simulink model "simulink_tirocinio3"  (R2021a)
settings: Solver=VariableStepAuto  StartTime=0.0  StopTime=100  RelTol=1e-3
values from neighbouring files (symbols this model uses):
  A = [lambda_1 0; 0 lambda_2]    [tirocinio1.m]    (also in tirocinio2.m = [0 1; gamma_1 gamma_2]; tirocinio3_complessiconiugati.m = [0 0 1 0; 0 0 0 1; -k_m/m1_m k_m/m1_m -c_m/m1_m c_m/m1_m; k_; tirocinio3_immaginari_puri.m = [0 0 1 0; 0 0 0 1; -k_m/m1_m k_m/m1_m -c_m/m1_m c_m/m1_m; k_; tirocinio3_reali.m = [0 0 1 0; 0 0 0 1; -k_m/m1_m k_m/m1_m -c_m/m1_m c_m/m1_m; k_)
  A_n = [0 0 1 0; 0 0 0 1; -k/m1 k/m1 -c/m1 c/m1; k/m2 -k/m2 c/m2 -c/m2]    [tirocinio3_complessiconiugati.m]    (also in tirocinio3_immaginari_puri.m; tirocinio3_reali.m; tirocinio4_rampa.m; tirocinio4_sinusoide.m)
  B = [1; 1]    [tirocinio1.m]    (also in tirocinio2.m = [0; 1]; tirocinio3_complessiconiugati.m = [0; 0; 1/m1_m; 0]; tirocinio3_immaginari_puri.m = [0; 0; 1/m1_m; 0]; tirocinio3_reali.m = [0; 0; 1/m1_m; 0])
  B_n = [0; 0; 1/m1; 0]    [tirocinio3_complessiconiugati.m]    (also in tirocinio3_immaginari_puri.m; tirocinio3_reali.m; tirocinio4_rampa.m; tirocinio4_sinusoide.m)
  C = [0, 0; 0 0]    [tirocinio2.m]    (also in tirocinio3_complessiconiugati.m = [1 0 0 0]; tirocinio3_immaginari_puri.m = [1 0 0 0]; tirocinio3_reali.m = [1 0 0 0]; tirocinio4_rampa.m = [1 0 0 0])
  csi0 = [0;0;0;0]    [tirocinio3_complessiconiugati.m]    (also in tirocinio3_immaginari_puri.m; tirocinio3_reali.m)
  d = 0    [tirocinio3_complessiconiugati.m]    (also in tirocinio3_immaginari_puri.m; tirocinio3_reali.m)
  H = A-V*C    [tirocinio3_complessiconiugati.m]    (also in tirocinio3_immaginari_puri.m; tirocinio3_reali.m)
  M = [0; 0; 0; 1/m2_m]    [tirocinio3_complessiconiugati.m]    (also in tirocinio3_immaginari_puri.m; tirocinio3_reali.m; tirocinio4_rampa.m = 2; tirocinio4_sinusoide.m = 1)
  M_n = [0; 0; 0; 1/m2]    [tirocinio3_complessiconiugati.m]    (also in tirocinio3_immaginari_puri.m; tirocinio3_reali.m)
  np = 0    [tirocinio3_complessiconiugati.m]    (also in tirocinio3_immaginari_puri.m; tirocinio3_reali.m)
  R = B-V*D    [tirocinio3_complessiconiugati.m]    (also in tirocinio3_immaginari_puri.m; tirocinio3_reali.m)
  V = -Fd'    [tirocinio3_complessiconiugati.m]    (also in tirocinio3_immaginari_puri.m; tirocinio3_reali.m; tirocinio4_rampa.m = -F_d'; tirocinio4_sinusoide.m = -F_d')
  x0 = [0;2;0;0]    [tirocinio3_complessiconiugati.m]    (also in tirocinio3_immaginari_puri.m; tirocinio3_reali.m = [1;10;3;2]; tirocinio4_rampa.m = [0; 2; 0; 0]; tirocinio4_sinusoide.m = [0;0;0;0])
libraries: simulink x2
settings Model: Creator=Valentina  LastModifiedBy=Valentina

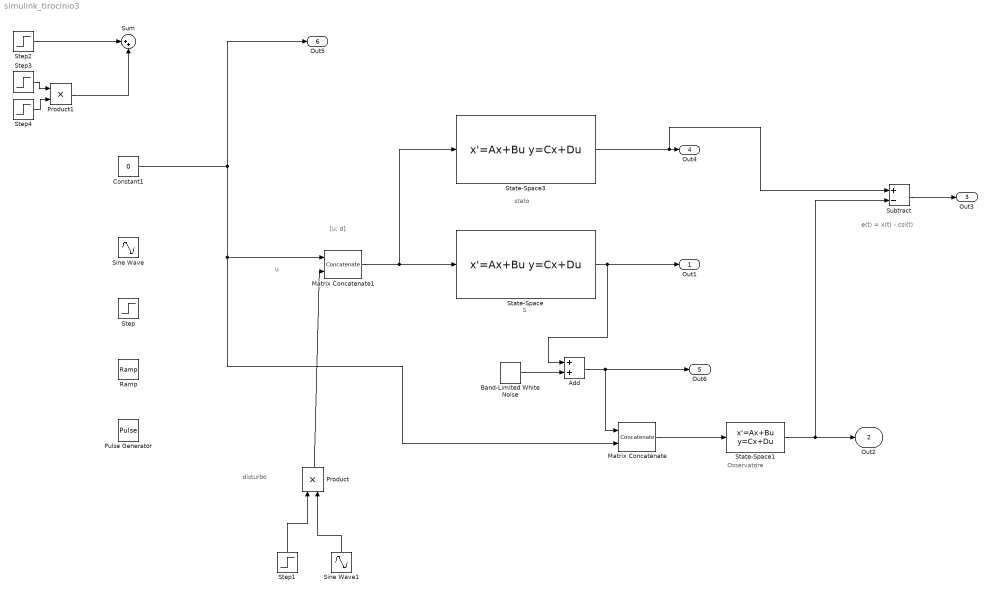
== system simulink_tirocinio3 ==
  note: [u; d]
  note: u
  note: disturbo
  note: e(t) = x(t) - csi(t)
  note: stato
  note: Osservatore
  note: S
  Add : Sum
  Band-Limited White Noise : simulink/Sources/Band-Limited White Noise  Cov=[np]  Ts=0.1  seed=[23341]
  Constant1 : Constant  Value=0
  Matrix Concatenate : Concatenate  Mode=Multidimensional array
  Matrix Concatenate1 : Concatenate  Mode=Multidimensional array
  Product : Product
  Product1 : Product
  Pulse Generator : DiscretePulseGenerator  PulseType=Time based  Amplitude=2  Period=100  PulseWidth=5
  Ramp : simulink/Sources/Ramp  slope=0.01  start=5  InitialOutput=0
  Sine Wave : Sin  SampleTime=0
  Sine Wave1 : Sin  Amplitude=d  SampleTime=0
  State-Space : StateSpace  A=A  B=[B M]  C=C  D=[0 0]  InitialCondition=x0  ParameterTunability=Unconstrained
  State-Space1 : StateSpace  A=H  B=[V R]  C=eye(4)  D=[0 0; 0 0; 0 0; 0 0]  InitialCondition=csi0
  State-Space3 : StateSpace  A=A_n  B=[B_n M_n]  C=eye(4)  D=[0 0;0 0;0 0;0 0]  InitialCondition=x0  ParameterTunability=Unconstrained
  Step : Step  Time=3  Before=2  After=0  SampleTime=0
  Step1 : Step  Time=15  Before=1  After=0  SampleTime=0
  Step2 : Step  Time=5  Before=5  After=0  SampleTime=0
  Step3 : Step  Time=10  After=-5  SampleTime=0
  Step4 : Step  Time=15  Before=1  After=0  SampleTime=0
  Subtract : Sum  Inputs=+-
  Sum : Sum  Inputs=|++
  Out1 : Outport  SignalName=y(t)
  Out2 : Outport  Port=2  SignalName=csi(t)
  Out3 : Outport  Port=3  SignalName=e(t)
  Out4 : Outport  Port=4  SignalName=x(t)
  Out6 : Outport  Port=5  SignalName=yd(t)
  Out5 : Outport  Port=6  SignalName=ingresso
  wires:
  Matrix Concatenate1/1 -> State-Space3/1, State-Space/1
  State-Space/1 -> Add/1, Out1/1
  Matrix Concatenate/1 -> State-Space1/1
  State-Space1/1 -> Subtract/2, Out2/1
  State-Space3/1 -> Subtract/1, Out4/1
  Subtract/1 -> Out3/1
  Sine Wave1/1 -> Product/2
  Step1/1 -> Product/1
  Constant1/1 -> Matrix Concatenate/2, Matrix Concatenate1/1, Out5/1
  Product/1 -> Matrix Concatenate1/2
  Band-Limited White Noise/1 -> Add/2
  Add/1 -> Out6/1, Matrix Concatenate/1
  Step3/1 -> Product1/1
  Step4/1 -> Product1/2
  Step2/1 -> Sum/1
  Product1/1 -> Sum/2
